simulink model "variacion_theta"  (R2026a)
settings: Solver=VariableStepAuto
values from neighbouring files (symbols this model uses):
  K = cambio_y / delta_u    [Taller_1_Identificacion_grafica_de_sistemas_FOTD.m]
  t_escalon = t(idx_escalon + 1)    [Taller_1_Identificacion_grafica_de_sistemas_FOTD.m]
  tau_analitico = 1.5 * (t_63_relativo - t_28_relativo)    [Taller_1_Identificacion_grafica_de_sistemas_FOTD.m]
  theta_analitico = t_63_relativo - tau_analitico    [Taller_1_Identificacion_grafica_de_sistemas_FOTD.m]
settings Model: Creator=Daniel  LastModifiedBy=Daniel

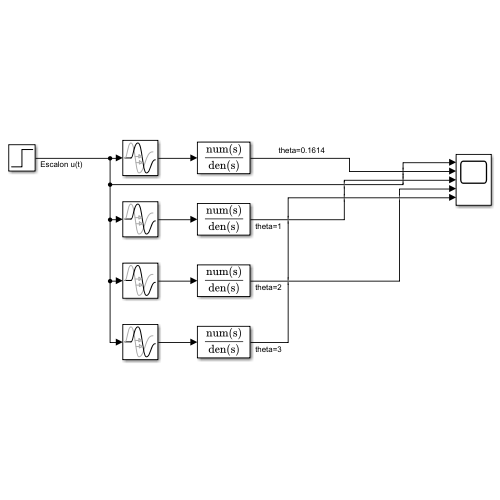
[thumbnail: Simulink's stored preview of the top-level diagram]
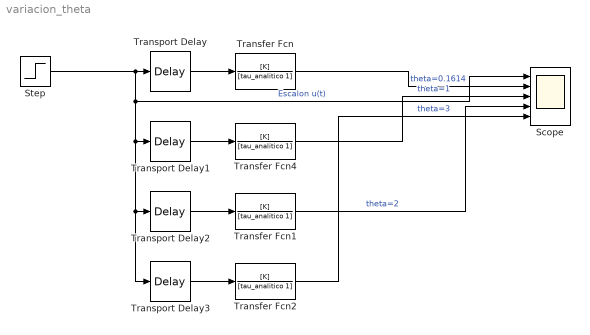
== system variacion_theta ==
  Scope : Scope  NumInputPorts=5
      settings: Title=Respuesta del Modelo Analítico  ActiveDisplayYMinimum=-0.4882625489147906  ActiveDisplayYMaximum=2.634836077109187  YLabel=Amplitud
  Step : Step  Time=t_escalon  FinalValue=1.5  SampleTime=0
  Transfer Fcn{,1..2,4} (4 alike) : TransferFcn  Numerator=[K]  Denominator=[tau_analitico 1]
  Transport Delay : TransportDelay  DelayTime=theta_analitico
  Transport Delay1 : TransportDelay
  Transport Delay2 : TransportDelay  DelayTime=2
  Transport Delay3 : TransportDelay  DelayTime=3
  wires:
  Transfer Fcn1/1 -> Scope/4  "theta=2"
  Transfer Fcn4/1 -> Scope/3  "theta=1"
  Transfer Fcn2/1 -> Scope/5  "theta=3"
  Step/1 -> Transport Delay3/1, Transport Delay2/1, Transport Delay1/1, Scope/1, Transport Delay/1  "Escalon u(t)"
  Transfer Fcn/1 -> Scope/2  "theta=0.1614"
  Transport Delay/1 -> Transfer Fcn/1
  Transport Delay1/1 -> Transfer Fcn4/1
  Transport Delay2/1 -> Transfer Fcn1/1
  Transport Delay3/1 -> Transfer Fcn2/1
